simulink library "aerosimlib"  (Simulink 5.0)
values from neighbouring files (symbols this model uses):
  stdatm = [0 100 200 300 400 500 600 700 800 900 1000 1100 ... (4305 elements, 861x5)]    [stdatm.mat]
undefined symbols (not defined in the file or in its folder): AlphaBnd, b, BetaBnd, CDda, CDde, CDdf, CDdr, CDM, CDmin, CGempty, CGgross, CL0, CLa, CLalphadot, Clbeta, Clda, CLde, CLdf, Cldr, CLM, CLmind, Clp, CLq, Clr, Cm0, Cma, Cmalphadot, Cmde, Cmdf, CmM, Cmq, Cnbeta, Cnda, Cndr, Cnp, Cnr, CP, CT, CYbeta, CYda, CYdr, CYp, CYr, Displacement, dmy, Engine, EulerIni, FuelFlow, FuelIni, J, Jempty, Jeng, Jgross, Jprop, MAC, MAP, MAPLim, MassIni, MaxPower, mempty ... (+25)
libraries: aerosimlib x350, simulink3 x41
(part 7 of 10)

== system aerosimlib/FlightGear-Compatible/Complete Aircraft/CESSNA-182 ==
  Control : Inport  PortDimensions=[8 1]
  Wind : Inport  Port=2  PortDimensions=[3 1]
  RST : Inport  Port=3  PortDimensions=1
  Aerodynamics : Subsystem
  Aircraft Inertia : Subsystem
  Atmosphere : aerosimlib/FlightGear-Compatible/Complete Aircraft/CESSNA-172/Atmosphere  SimViewingDevice=off
      settings: Permissions=ReadWrite  RTWFcnNameOpts=Auto  RTWFileNameOpts=Auto
  Demux : Demux  Outputs=8
  Demux1 : Demux  Outputs=3
  Earth : Subsystem
  Equations of Motion : Subsystem
  F/m : Product  Inputs=*/  SaturateOnIntegerOverflow=on  InputSameDT=on
  FG Piston Engine +  Variable-Pitch Prop : aerosimlib/FlightGear-Compatible/Propulsion/FG Piston Engine +  Variable-Pitch Prop  Eng=AC.Propulsion.Engine{1}  Thr=AC.Propulsion.Thruster{1}  pSL=101325  TSL=288.15  OmegaIni=OmegaIni
  Mux : Mux
  Mux1 : Mux
  Sum1 : Sum  SaturateOnIntegerOverflow=on  InputSameDT=on
  Sum2 : Sum  SaturateOnIntegerOverflow=on  InputSameDT=on
  rad/s 2 RPM : aerosimlib/Unit Conversion/Angular velocity/rad//s 2 RPM
  TAS : Outport
  AOA : Outport  Port=2
  Position : Outport  Port=3
  Attitude : Outport  Port=4
  Rates : Outport  Port=5
  Aero : Outport  Port=6
  Prop : Outport  Port=7
  Engine : Outport  Port=8
  RPM : Outport  Port=9
  wires:
  Demux/8 -> Mux1/4
  rad/s 2 RPM/1 -> RPM/1
  FG Piston Engine +  Variable-Pitch Prop/3 -> rad/s 2 RPM/1
  FG Piston Engine +  Variable-Pitch Prop/5 -> Engine/1
  FG Piston Engine +  Variable-Pitch Prop/6 -> Prop/1
  Aerodynamics/3(AeroCoeff) -> Aero/1
  Equations of Motion/7(Euler) -> Attitude/1
  Demux1/3 -> AOA/1
  Demux1/1 -> TAS/1
  Equations of Motion/6(DCM) -> Atmosphere/6
  Equations of Motion/1(VelB) -> Aerodynamics/2(VelB), Atmosphere/4
  Equations of Motion/3(Rates) -> Rates/1, Aerodynamics/4(Rates)
  Earth/2(AGL) -> Aerodynamics/8(AGL), Atmosphere/2
  Earth/1(MSL) -> Atmosphere/1
  Earth/3(AConGnd) -> Equations of Motion/6(AConGnd)
  Earth/6(Gravity) -> Equations of Motion/5(Gravity)
  Earth/4(Rearth) -> Equations of Motion/4(Rearth)
  Equations of Motion/5(Pos) -> Position/1, Earth/1(Position)
  Aircraft Inertia/3(Inertia) -> Equations of Motion/3(Inertia)
  F/m/1 -> Equations of Motion/1(Accel)
  Aircraft Inertia/2(CG) -> FG Piston Engine +  Variable-Pitch Prop/6, Aerodynamics/9(CGpos)
  Aircraft Inertia/1(Mass) -> F/m/2
  FG Piston Engine +  Variable-Pitch Prop/4 -> Aircraft Inertia/1(FuelFlow)
  RST/1 -> Aircraft Inertia/2(RST), Equations of Motion/7(RST), FG Piston Engine +  Variable-Pitch Prop/7
  Aerodynamics/4(VelW) -> Demux1/1, FG Piston Engine +  Variable-Pitch Prop/5, Atmosphere/5
  Atmosphere/2 -> FG Piston Engine +  Variable-Pitch Prop/3
  Atmosphere/1 -> FG Piston Engine +  Variable-Pitch Prop/2
  Atmosphere/5 -> Aerodynamics/3(WindB)
  Atmosphere/6 -> Aerodynamics/5(WindRates)
  Wind/1 -> Atmosphere/3
  Atmosphere/4 -> Aerodynamics/7(a)
  Atmosphere/3 -> FG Piston Engine +  Variable-Pitch Prop/4, Aerodynamics/6(rho)
  Mux1/1 -> FG Piston Engine +  Variable-Pitch Prop/1
  Mux/1 -> Aerodynamics/1(Control)
  Control/1 -> Demux/1
  Demux/7 -> Mux1/3
  Demux/6 -> Mux1/2
  Demux/5 -> Mux1/1
  Demux/4 -> Mux/4
  Demux/3 -> Mux/3
  Demux/2 -> Mux/2
  Demux/1 -> Mux/1
  FG Piston Engine +  Variable-Pitch Prop/2 -> Sum1/2
  Sum2/1 -> F/m/1
  Sum1/1 -> Equations of Motion/2(Moment)
  Aerodynamics/1(Faero) -> Sum2/1
  Aerodynamics/2(Maero) -> Sum1/1
  FG Piston Engine +  Variable-Pitch Prop/1 -> Sum2/2

== system aerosimlib/FlightGear-Compatible/Complete Aircraft/CESSNA-310 ==
  Control : Inport  PortDimensions=[12 1]
  Gear : Inport  Port=2  PortDimensions=1
  Wind : Inport  Port=3  PortDimensions=[3 1]
  RST : Inport  Port=4  PortDimensions=1
  Aerodynamics : Subsystem
  Aircraft Inertia : Subsystem
  Atmosphere : aerosimlib/FlightGear-Compatible/Complete Aircraft/CESSNA-172/Atmosphere  SimViewingDevice=off
      settings: Permissions=ReadWrite  RTWFcnNameOpts=Auto  RTWFileNameOpts=Auto
  Demux : Demux  Outputs=3
  Demux1 : Demux  Outputs=3
  Earth : Subsystem
  Equations of Motion : Subsystem
  F/m : Product  Inputs=*/  SaturateOnIntegerOverflow=on  InputSameDT=on
  Left Engine : aerosimlib/FlightGear-Compatible/Propulsion/FG Piston Engine +  Variable-Pitch Prop  Eng=AC.Propulsion.Engine{1}  Thr=AC.Propulsion.Thruster{1}  pSL=101325  TSL=288.15  OmegaIni=OmegaIni(1)
  Right Engine : aerosimlib/FlightGear-Compatible/Propulsion/FG Piston Engine +  Variable-Pitch Prop  Eng=AC.Propulsion.Engine{2}  Thr=AC.Propulsion.Thruster{2}  pSL=101325  TSL=288.15  OmegaIni=OmegaIni(2)
  Sum : Sum  Orientation=left  Inputs=|++  SaturateOnIntegerOverflow=on  InputSameDT=on
  Sum1 : Sum  Inputs=+++  SaturateOnIntegerOverflow=on  InputSameDT=on
  Sum2 : Sum  Inputs=+++  SaturateOnIntegerOverflow=on  InputSameDT=on
  rad/s 2 RPM : aerosimlib/Unit Conversion/Angular velocity/rad//s 2 RPM
  rad/s 2 RPM1 : aerosimlib/Unit Conversion/Angular velocity/rad//s 2 RPM
  TAS : Outport
  AOA : Outport  Port=2
  Position : Outport  Port=3
  Attitude : Outport  Port=4
  Rates : Outport  Port=5
  Aero : Outport  Port=6
  PropL : Outport  Port=7
  EngineL : Outport  Port=8
  RPML : Outport  Port=9
  PropR : Outport  Port=10
  EngineR : Outport  Port=11
  RPMR : Outport  Port=12
  wires:
  Gear/1 -> Aerodynamics/10(Gear)
  Demux/1 -> Aerodynamics/1(Control)
  Earth/1(MSL) -> Atmosphere/1
  Equations of Motion/6(DCM) -> Atmosphere/6
  Earth/2(AGL) -> Aerodynamics/8(AGL), Atmosphere/2
  Atmosphere/4 -> Aerodynamics/7(a)
  Atmosphere/6 -> Aerodynamics/5(WindRates)
  Atmosphere/5 -> Aerodynamics/3(WindB)
  Equations of Motion/1(VelB) -> Aerodynamics/2(VelB), Atmosphere/4
  rad/s 2 RPM1/1 -> RPMR/1
  Right Engine/5 -> EngineR/1
  Right Engine/6 -> PropR/1
  rad/s 2 RPM/1 -> RPML/1
  Left Engine/6 -> PropL/1
  Left Engine/5 -> EngineL/1
  Right Engine/3 -> rad/s 2 RPM1/1
  Left Engine/3 -> rad/s 2 RPM/1
  Right Engine/2 -> Sum2/2
  Left Engine/2 -> Sum2/3
  Aerodynamics/2(Maero) -> Sum2/1
  Sum2/1 -> Equations of Motion/2(Moment)
  Right Engine/1 -> Sum1/2
  Left Engine/1 -> Sum1/3
  Aircraft Inertia/1(Mass) -> F/m/2
  Sum1/1 -> F/m/1
  F/m/1 -> Equations of Motion/1(Accel)
  Sum/1 -> Aircraft Inertia/1(FuelFlow)
  Left Engine/4 -> Sum/2
  Right Engine/4 -> Sum/1
  Atmosphere/3 -> Aerodynamics/6(rho), Right Engine/4, Left Engine/4
  Atmosphere/2 -> Right Engine/3, Left Engine/3
  Atmosphere/1 -> Right Engine/2, Left Engine/2
  Demux/3 -> Right Engine/1
  Demux/2 -> Left Engine/1
  Wind/1 -> Atmosphere/3
  Aerodynamics/3(AeroCoeff) -> Aero/1
  Equations of Motion/7(Euler) -> Attitude/1
  Demux1/3 -> AOA/1
  Demux1/1 -> TAS/1
  Equations of Motion/3(Rates) -> Rates/1, Aerodynamics/4(Rates)
  Earth/3(AConGnd) -> Equations of Motion/6(AConGnd)
  Earth/6(Gravity) -> Equations of Motion/5(Gravity)
  Earth/4(Rearth) -> Equations of Motion/4(Rearth)
  Equations of Motion/5(Pos) -> Position/1, Earth/1(Position)
  Aircraft Inertia/3(Inertia) -> Equations of Motion/3(Inertia)
  Aircraft Inertia/2(CG) -> Left Engine/6, Aerodynamics/9(CGpos), Right Engine/6
  Aerodynamics/1(Faero) -> Sum1/1
  RST/1 -> Right Engine/7, Left Engine/7, Aircraft Inertia/2(RST), Equations of Motion/7(RST)
  Aerodynamics/4(VelW) -> Right Engine/5, Left Engine/5, Atmosphere/5, Demux1/1
  Control/1 -> Demux/1

== system aerosimlib/FlightGear-Compatible/Inertia/Empty Aircraft ==
  ACMass : Constant  Value=Metrics.EmptyWeight
  CG Location : Constant  Value=Metrics.CGLoc
  Moments of Inertia : Constant  Value=[Metrics.InertiaX Metrics.InertiaY Metrics.InertiaZ Metrics.InertiaXZ]
  Mass : Outport
  CG : Outport  Port=2
  Inertia : Outport  Port=3
  wires:
  ACMass/1 -> Mass/1
  CG Location/1 -> CG/1
  Moments of Inertia/1 -> Inertia/1

== system aerosimlib/FlightGear-Compatible/Inertia/Point Mass ==
  J1 : Product  SaturateOnIntegerOverflow=on  InputSameDT=on
  J2 : Product  SaturateOnIntegerOverflow=on  InputSameDT=on
  J3 : Product  SaturateOnIntegerOverflow=on  InputSameDT=on
  Jxz : Product  Inputs=3  SaturateOnIntegerOverflow=on  InputSameDT=on
  M : Constant  Value=PointMass(1)
  Math Function1 : Math  Operator=square
  Math Function2 : Math  Operator=square
  Math Function3 : Math  Operator=square
  Mux : Mux  Inputs=3
  Mux1 : Mux
  Sum : Sum  SaturateOnIntegerOverflow=on  InputSameDT=on
  Sum1 : Sum  SaturateOnIntegerOverflow=on  InputSameDT=on
  Sum2 : Sum  SaturateOnIntegerOverflow=on  InputSameDT=on
  x pos : Constant  Value=PointMass(2)
  y pos : Constant  Value=PointMass(3)
  z pos : Constant  Value=PointMass(4)
  Mass : Outport
  CG : Outport  Port=2
  Inertia : Outport  Port=3
  wires:
  J3/1 -> Mux1/3
  J2/1 -> Mux1/2
  J1/1 -> Mux1/1
  Mux1/1 -> Inertia/1
  Jxz/1 -> Mux1/4
  Mux/1 -> CG/1
  Sum/1 -> J3/2
  Sum2/1 -> J2/2
  Sum1/1 -> J1/2
  Math Function3/1 -> Sum2/2, Sum1/2
  Math Function2/1 -> Sum1/1, Sum/2
  Math Function1/1 -> Sum2/1, Sum/1
  z pos/1 -> Math Function3/1, Mux/3, Jxz/3
  y pos/1 -> Mux/2, Math Function2/1
  x pos/1 -> Mux/1, Jxz/2, Math Function1/1
  M/1 -> Mass/1, J1/1, J2/1, J3/1, Jxz/1

== system aerosimlib/FlightGear-Compatible/Propulsion/Engine ==
  Piston : Subsystem

== system aerosimlib/FlightGear-Compatible/Propulsion/FG Piston Engine +  Fixed-Pitch Prop ==
  Control : Inport  PortDimensions=[3 1]  DataType=double
  p : Inport  Port=2  PortDimensions=1  DataType=double
  T : Inport  Port=3  PortDimensions=1  DataType=double
  rho : Inport  Port=4  PortDimensions=1  DataType=double
  WindAxesVel : Inport  Port=5  PortDimensions=[3 1]
  CGpos : Inport  Port=6  PortDimensions=[3 1]
  RST : Inport  Port=7  PortDimensions=1  DataType=double
  ChSign : Gain  Gain=-Thr.Sense  SaturateOnIntegerOverflow=on
  Demux : Demux  Outputs=3
  Demux1 : Demux  Outputs=3
  Engine speed Integrator : Integrator  ExternalReset=rising  InitialCondition=OmegaIni  LimitOutput=on  LowerSaturationLimit=0
  FG Fixed-Pitch Propeller : aerosimlib/FlightGear-Compatible/Propulsion/Thruster/Propeller/FG Fixed-Pitch Propeller  Thr=Thr
  FG Piston Engine : aerosimlib/FlightGear-Compatible/Propulsion/Engine/Piston/FG Piston Engine  Eng=Eng  pSL=pSL  TSL=TSL
  M/J : Product  Inputs=*/  SaturateOnIntegerOverflow=on  InputSameDT=on
  Mux : Mux  Inputs=3
  Mux1 : Mux  Inputs=3
  Mux2 : Mux  Inputs=5
  Propeller  moment of inertia : Constant  Value=Thr.Param.Inertia
  Sum : Sum  Inputs=|+-  SaturateOnIntegerOverflow=on  InputSameDT=on
  Sum1 : Sum  SaturateOnIntegerOverflow=on  InputSameDT=on
  Sum2 : Sum  Inputs=|++  SaturateOnIntegerOverflow=on  InputSameDT=on
  Terminator : Terminator
  Terminator1 : Terminator
  Zero : Constant  Value=0
  r x F : aerosimlib/Math/Cross Product
  r_prop : Constant  Value=Thr.Loc
  Fprop : Outport
  Mprop : Outport  Port=2
  Omega : Outport  Port=3
  FuelFlow : Outport  Port=4
  EngCoeff : Outport  Port=5
  PropCoeff : Outport  Port=6
  wires:
  Control/1 -> Demux/1
  WindAxesVel/1 -> Demux1/1
  Demux1/2 -> Terminator/1
  Demux1/3 -> Terminator1/1
  Demux1/1 -> FG Fixed-Pitch Propeller/1
  rho/1 -> FG Piston Engine/6, FG Fixed-Pitch Propeller/2
  Propeller  moment of inertia/1 -> M/J/2
  FG Fixed-Pitch Propeller/2 -> Sum1/2
  Sum1/1 -> M/J/1
  M/J/1 -> Engine speed Integrator/1
  RST/1 -> Engine speed Integrator/2
  Engine speed Integrator/1 -> FG Piston Engine/3, FG Fixed-Pitch Propeller/3, Omega/1
  Zero/1 -> Mux/2, Mux/3, Mux1/3, Mux1/2
  FG Fixed-Pitch Propeller/1 -> Mux/1
  ChSign/1 -> Mux1/1
  FG Fixed-Pitch Propeller/3 -> PropCoeff/1
  Demux/1 -> FG Piston Engine/1
  Demux/2 -> FG Piston Engine/2
  p/1 -> FG Piston Engine/4
  T/1 -> FG Piston Engine/5
  FG Piston Engine/6 -> ChSign/1, Sum1/1
  FG Piston Engine/1 -> Mux2/1
  FG Piston Engine/2 -> Mux2/2
  FG Piston Engine/3 -> Mux2/3, FuelFlow/1
  FG Piston Engine/4 -> Mux2/4
  FG Piston Engine/5 -> Mux2/5
  Mux2/1 -> EngCoeff/1
  r_prop/1 -> Sum/1
  CGpos/1 -> Sum/2
  Sum/1 -> r x F/1
  Mux/1 -> r x F/2, Fprop/1
  Mux1/1 -> Sum2/1
  r x F/1 -> Sum2/2
  Sum2/1 -> Mprop/1

== system aerosimlib/FlightGear-Compatible/Propulsion/FG Piston Engine +  Variable-Pitch Prop ==
  Control : Inport  PortDimensions=[4 1]  DataType=double
  p : Inport  Port=2  PortDimensions=1  DataType=double
  T : Inport  Port=3  PortDimensions=1  DataType=double
  rho : Inport  Port=4  PortDimensions=1  DataType=double
  WindAxesVel : Inport  Port=5  PortDimensions=[3 1]
  CGpos : Inport  Port=6  PortDimensions=[3 1]
  RST : Inport  Port=7  PortDimensions=1  DataType=double
  ChSign : Gain  Gain=-Thr.Sense  SaturateOnIntegerOverflow=on
  Demux : Demux
  Demux1 : Demux  Outputs=3
  Engine speed Integrator : Integrator  ExternalReset=rising  InitialCondition=OmegaIni  LimitOutput=on  LowerSaturationLimit=0
  FG Piston Engine : aerosimlib/FlightGear-Compatible/Propulsion/Engine/Piston/FG Piston Engine  Eng=Eng  pSL=pSL  TSL=TSL
  FG Variable-Pitch Propeller : aerosimlib/FlightGear-Compatible/Propulsion/Thruster/Propeller/FG Variable-Pitch Propeller  Thr=Thr
  M/J : Product  Inputs=*/  SaturateOnIntegerOverflow=on  InputSameDT=on
  Mux : Mux  Inputs=3
  Mux1 : Mux  Inputs=3
  Mux2 : Mux  Inputs=5
  Propeller  moment of inertia : Constant  Value=Thr.Param.Inertia
  Sum : Sum  Inputs=|+-  SaturateOnIntegerOverflow=on  InputSameDT=on
  Sum1 : Sum  SaturateOnIntegerOverflow=on  InputSameDT=on
  Sum2 : Sum  Inputs=|++  SaturateOnIntegerOverflow=on  InputSameDT=on
  Terminator : Terminator
  Terminator1 : Terminator
  Zero : Constant  Value=0
  r x F : aerosimlib/Math/Cross Product
  r_prop : Constant  Value=Thr.Loc
  Fprop : Outport
  Mprop : Outport  Port=2
  Omega : Outport  Port=3
  FuelFlow : Outport  Port=4
  EngCoeff : Outport  Port=5
  PropCoeff : Outport  Port=6
  wires:
  Demux/4 -> FG Variable-Pitch Propeller/4
  Control/1 -> Demux/1
  WindAxesVel/1 -> Demux1/1
  Demux1/2 -> Terminator/1
  Demux1/3 -> Terminator1/1
  Demux1/1 -> FG Variable-Pitch Propeller/1
  rho/1 -> FG Variable-Pitch Propeller/2, FG Piston Engine/6
  Propeller  moment of inertia/1 -> M/J/2
  FG Variable-Pitch Propeller/2 -> Sum1/2
  Sum1/1 -> M/J/1
  M/J/1 -> Engine speed Integrator/1
  RST/1 -> Engine speed Integrator/2
  Engine speed Integrator/1 -> FG Variable-Pitch Propeller/3, FG Piston Engine/3, Omega/1
  Zero/1 -> Mux/2, Mux/3, Mux1/3, Mux1/2
  FG Variable-Pitch Propeller/1 -> Mux/1
  ChSign/1 -> Mux1/1
  FG Variable-Pitch Propeller/3 -> PropCoeff/1
  Demux/1 -> FG Piston Engine/1
  Demux/2 -> FG Piston Engine/2
  p/1 -> FG Piston Engine/4
  T/1 -> FG Piston Engine/5
  FG Piston Engine/6 -> ChSign/1, Sum1/1
  FG Piston Engine/1 -> Mux2/1
  FG Piston Engine/2 -> Mux2/2
  FG Piston Engine/3 -> Mux2/3, FuelFlow/1
  FG Piston Engine/4 -> Mux2/4
  FG Piston Engine/5 -> Mux2/5
  Mux2/1 -> EngCoeff/1
  r_prop/1 -> Sum/1
  CGpos/1 -> Sum/2
  Sum/1 -> r x F/1
  Mux/1 -> r x F/2, Fprop/1
  Mux1/1 -> Sum2/1
  r x F/1 -> Sum2/2
  Sum2/1 -> Mprop/1

== system aerosimlib/FlightGear-Compatible/Propulsion/Tank ==
  Fuel Tank : Subsystem  mask(Fuel Tank){MassIni=MassIni, Tank=Tank}
      mask prompts: MassIni "Initial mass:"; Tank "Tank structure:"
      mask help: The block integrates fuel flow to compute the tank inertia parameters.
      mask init:
      | if MassIni > Tank.Capacity
      | 	% Limit initial mass to tank capacity
      | 	MassIni = Tank.Capacity;
      | end
      mask Help:
      | The block integrates fuel flow to compute the tank inertia parameters.
      | <P><B>Inputs:</B>
      | <LI>MassFlow = the current propellant mass flow (positive for propellant flowing out of the tank, negative otherwise)</LI>
      | <LI>RST = the flow integrator reset flag (integrator resets on rising edge)</LI>
      | </P>
      | <P><B>Outputs:</B>
      | <LI>Mass = the current mass of the propellant in the tank</LI>
      | <LI>CG = the tank CG location, in aircraft coordinates</LI>
      | <LI>Inertia = the tank moments of inertia [Jx Jy Jz Jxz]</LI>
      | </P>
      | <P><B>Parameters:</B>
      | <LI>Initial mass = the initial mass of propellant in the tank</LI>
      | <LI>Tank structure = the Matlab tank structure, part of the aircraft structure</LI>
      | </P>

== system aerosimlib/FlightGear-Compatible/Propulsion/Thruster ==
  Propeller : Subsystem

== system aerosimlib/Math/Normalization/Vector norm ==
  Vec : Inport
  Dot Product : simulink3/Math/Dot Product
  Math Function : Math  Operator=sqrt
  Mag : Outport
  wires:
  Math Function/1 -> Mag/1
  Dot Product/1 -> Math Function/1
  Vec/1 -> Dot Product/2, Dot Product/1

== system aerosimlib/Math/Zero Offset/Non-zero Sign ==
  In : Inport
  One : Constant
  Relational Operator : RelationalOperator  Operator===  InputSameDT=on
  Sign : Signum
  Switch : Switch  Threshold=1  SaturateOnIntegerOverflow=on  InputSameDT=on
  Zero : Constant  Value=0
  Out : Outport
  wires:
  Zero/1 -> Relational Operator/2
  In/1 -> Relational Operator/1, Sign/1
  Relational Operator/1 -> Switch/2
  One/1 -> Switch/1
  Sign/1 -> Switch/3
  Switch/1 -> Out/1

== system aerosimlib/Propulsion/Piston Engine/Intake ==
  Thr : Inport  PortDimensions=1  DataType=double
  p : Inport  Port=2  PortDimensions=1  DataType=double
  Get MAP : Product  SaturateOnIntegerOverflow=on  InputSameDT=on
  MAP min : Constant  Value=MAPmin
  Saturation : Saturate  UpperLimit=inf  LowerLimit=MAPmin
  Sum : Sum  Inputs=|+-  SaturateOnIntegerOverflow=on  InputSameDT=on
  Sum1 : Sum  Inputs=|++  SaturateOnIntegerOverflow=on  InputSameDT=on
  kPa : Gain  Gain=1/1000  SaturateOnIntegerOverflow=on
  MAP : Outport
  wires:
  Saturation/1 -> MAP/1
  p/1 -> kPa/1
  Thr/1 -> Get MAP/1
  MAP min/1 -> Sum/2, Sum1/2
  kPa/1 -> Sum/1
  Sum/1 -> Get MAP/2
  Get MAP/1 -> Sum1/1
  Sum1/1 -> Saturation/1

== system aerosimlib/Sensors/Analog Sensors/A/D Converter ==
  Analog : Inport
  Count size in Volts : Product  Inputs=*/  SaturateOnIntegerOverflow=on  InputSameDT=on
  Max Counts : Constant  Value=2^Bits
  Max Volts : Constant  Value=MaxVolts
  Min Volts : Constant  Value=MinVolts
  Number of counts : Product  Inputs=*/  SaturateOnIntegerOverflow=on  InputSameDT=on
  Rounding Function : Rounding
  Saturation : Saturate  UpperLimit=2^Bits  LowerLimit=0
  Sum : Sum  Inputs=|+-  SaturateOnIntegerOverflow=on  InputSameDT=on
  Sum1 : Sum  Inputs=|+-  SaturateOnIntegerOverflow=on  InputSameDT=on
  Zero-Order Hold : ZeroOrderHold  SampleTime=tsamp
  Digital : Outport
  wires:
  Zero-Order Hold/1 -> Digital/1
  Saturation/1 -> Zero-Order Hold/1
  Max Volts/1 -> Sum/1
  Min Volts/1 -> Sum/2, Sum1/2
  Max Counts/1 -> Count size in Volts/2
  Sum/1 -> Count size in Volts/1
  Analog/1 -> Sum1/1
  Sum1/1 -> Number of counts/1
  Count size in Volts/1 -> Number of counts/2
  Number of counts/1 -> Rounding Function/1
  Rounding Function/1 -> Saturation/1

== system aerosimlib/Sensors/Analog Sensors/Analog Sensor ==
  Input : Inport  PortDimensions=1
  Bias Voltage : Constant  Value=BiasVolt
  Bias Point : Constant  Value=BiasPoint
  Scale Factor : Constant  Value=ScaleFactor
  Simple Sensor (2nd-order dynamics) : aerosimlib/Sensors/Generic Sensors/Simple Sensor (2nd-order dynamics)  MaxInput=Range(2)  MinInput=Range(1)  Bandwidth=Bandwidth  NoiseSeed=NoiseSeed  NoiseCov=NoiseCov  SampleTime=SampleTime
  Sum1 : Sum  Inputs=|++  SaturateOnIntegerOverflow=on  InputSameDT=on
  Sum2 : Sum  Inputs=|+-  SaturateOnIntegerOverflow=on  InputSameDT=on
  Unit conversion : Product  SaturateOnIntegerOverflow=on  InputSameDT=on
  Output : Outport
  wires:
  Simple Sensor (2nd-order dynamics)/1 -> Sum2/1
  Bias Point/1 -> Sum2/2
  Sum2/1 -> Unit conversion/1
  Scale Factor/1 -> Unit conversion/2
  Unit conversion/1 -> Sum1/1
  Bias Voltage/1 -> Sum1/2
  Sum1/1 -> Output/1
  Input/1 -> Simple Sensor (2nd-order dynamics)/1

== system aerosimlib/Sensors/Digital Sensors/GPS PV ==
  PVIn : Inport
  Altitude Measurement : aerosimlib/Sensors/Digital Sensors/Single GPS Measurement  ValIni=PosIni(3)  Lag=PosLag  TimeConst=TimeConst  seed=[32214]  Cov=VPosErr  T1=Trw
  Demux : Demux  Outputs=6
  Latitude Measurement : aerosimlib/Sensors/Digital Sensors/Single GPS Measurement  ValIni=PosIni(1)  Lag=PosLag  TimeConst=TimeConst  seed=[44123]  Cov=HPosErr/REarth  T1=Trw
  Longitude Measurement : aerosimlib/Sensors/Digital Sensors/Single GPS Measurement  ValIni=PosIni(2)  Lag=PosLag  TimeConst=TimeConst  seed=[11243]  Cov=HPosErr/REarth  T1=Trw
  Mux : Mux  Inputs=6
  V Down Measurement : aerosimlib/Sensors/Digital Sensors/Single GPS Measurement  ValIni=VelIni(3)  Lag=VelLag  TimeConst=TimeConst  seed=[21143]  Cov=VVelErr  T1=Trw
  V East Measurement : aerosimlib/Sensors/Digital Sensors/Single GPS Measurement  ValIni=VelIni(2)  Lag=VelLag  TimeConst=TimeConst  seed=[43321]  Cov=HVelErr  T1=Trw
  V North Measurement : aerosimlib/Sensors/Digital Sensors/Single GPS Measurement  ValIni=VelIni(1)  Lag=VelLag  TimeConst=TimeConst  seed=[12344]  Cov=HVelErr  T1=Trw
  PVOut : Outport
  wires:
  Demux/1 -> Latitude Measurement/1
  Demux/2 -> Longitude Measurement/1
  Demux/3 -> Altitude Measurement/1
  Demux/4 -> V North Measurement/1
  Demux/5 -> V East Measurement/1
  Demux/6 -> V Down Measurement/1
  PVIn/1 -> Demux/1
  Latitude Measurement/1 -> Mux/1
  Longitude Measurement/1 -> Mux/2
  Altitude Measurement/1 -> Mux/3
  V North Measurement/1 -> Mux/4
  V East Measurement/1 -> Mux/5
  V Down Measurement/1 -> Mux/6
  Mux/1 -> PVOut/1

== system aerosimlib/Sensors/Digital Sensors/Single GPS Measurement ==
  In : Inport
  Gauss-Markov  Process : aerosimlib/Sensors/Noise Correlation/Gauss-Markov  Process  beta=TimeConst  seed=seed  Var=Cov^2  T=T1
  Sum : Sum  Inputs=|++  SaturateOnIntegerOverflow=on  InputSameDT=on
  Transport Delay : TransportDelay  DelayTime=Lag  InitialInput=ValIni
  Out : Outport
  wires:
  Sum/1 -> Out/1
  Gauss-Markov  Process/1 -> Sum/2
  In/1 -> Transport Delay/1
  Transport Delay/1 -> Sum/1

== system aerosimlib/Sensors/Generic Sensors/Simple Sensor (1st-order dynamics) ==
  Input : Inport
  Random Walk : aerosimlib/Sensors/Noise Correlation/Random Walk  seed=NoiseSeed  Var=NoiseCov  T=SampleTime
  Saturation : Saturate  UpperLimit=MaxInput  LowerLimit=MinInput
  Sum : Sum  Inputs=|++  SaturateOnIntegerOverflow=on  InputSameDT=on
  Transfer Fcn : TransferFcn  Denominator=[Lag 1]
  Output : Outport
  wires:
  Sum/1 -> Output/1
  Random Walk/1 -> Sum/2
  Transfer Fcn/1 -> Sum/1
  Saturation/1 -> Transfer Fcn/1
  Input/1 -> Saturation/1

== system aerosimlib/Sensors/Generic Sensors/Simple Sensor (2nd-order dynamics) ==
  Input : Inport
  Random Walk : aerosimlib/Sensors/Noise Correlation/Random Walk  seed=NoiseSeed  Var=NoiseCov  T=SampleTime
  Saturation : Saturate  UpperLimit=MaxInput  LowerLimit=MinInput
  Sum : Sum  Inputs=|++  SaturateOnIntegerOverflow=on  InputSameDT=on
  Transfer Fcn : TransferFcn  Numerator=[wn^2]  Denominator=[1 2*zeta*wn wn^2]
  Output : Outport
  wires:
  Input/1 -> Saturation/1
  Saturation/1 -> Transfer Fcn/1
  Transfer Fcn/1 -> Sum/1
  Random Walk/1 -> Sum/2
  Sum/1 -> Output/1

== system aerosimlib/Sensors/Noise Correlation/Gauss-Markov  Process ==
  Gain : Gain  Orientation=left  Gain=1/beta  SaturateOnIntegerOverflow=on
  Integrator : Integrator
  Sum : Sum  Inputs=|+-  SaturateOnIntegerOverflow=on  InputSameDT=on
  White Noise : RandomNumber  Variance=Var  Seed=seed  SampleTime=T
  Out : Outport
  wires:
  Integrator/1 -> Out/1, Gain/1
  White Noise/1 -> Sum/1
  Sum/1 -> Integrator/1
  Gain/1 -> Sum/2

== system aerosimlib/Sensors/Noise Correlation/Random Walk ==
  Integrator : Integrator
  White Noise : RandomNumber  Variance=Var  Seed=seed  SampleTime=T
  Out : Outport
  wires:
  White Noise/1 -> Integrator/1
  Integrator/1 -> Out/1

== system aerosimlib/Unit Conversion/Angular position/deg 2 rad ==
  In : Inport
  Gain : Gain  Gain=pi/180  SaturateOnIntegerOverflow=on
  Out : Outport
  wires:
  Gain/1 -> Out/1
  In/1 -> Gain/1

== system aerosimlib/Unit Conversion/Angular position/rad 2 deg ==
  In : Inport
  Gain : Gain  Gain=180/pi  SaturateOnIntegerOverflow=on
  Out : Outport
  wires:
  In/1 -> Gain/1
  Gain/1 -> Out/1

== system aerosimlib/Unit Conversion/Angular velocity/RPM 2 rad/s ==
  In : Inport
  Gain : Gain  Gain=pi/30  SaturateOnIntegerOverflow=on
  Out : Outport
  wires:
  In/1 -> Gain/1
  Gain/1 -> Out/1

== system aerosimlib/Unit Conversion/Angular velocity/rad/s 2 RPM ==
  In : Inport
  Gain : Gain  Gain=30/pi  SaturateOnIntegerOverflow=on
  Out : Outport
  wires:
  Gain/1 -> Out/1
  In/1 -> Gain/1

== system aerosimlib/Unit Conversion/Distance/ft 2 m ==
  In : Inport
  Gain : Gain  Gain=0.3048  SaturateOnIntegerOverflow=on
  Out : Outport
  wires:
  In/1 -> Gain/1
  Gain/1 -> Out/1

== system aerosimlib/Unit Conversion/Distance/m 2 ft ==
  In : Inport
  Gain : Gain  Gain=1/0.3048  SaturateOnIntegerOverflow=on
  Out : Outport
  wires:
  Gain/1 -> Out/1
  In/1 -> Gain/1

== system aerosimlib/Unit Conversion/Distance/m 2 nm ==
  In : Inport
  Gain : Gain  Gain=1/1853.24496  SaturateOnIntegerOverflow=on
  Out : Outport
  wires:
  In/1 -> Gain/1
  Gain/1 -> Out/1

== system aerosimlib/Unit Conversion/Distance/nm 2 m ==
  In : Inport
  Gain : Gain  Gain=1853.24496  SaturateOnIntegerOverflow=on
  Out : Outport
  wires:
  Gain/1 -> Out/1
  In/1 -> Gain/1

== system aerosimlib/Unit Conversion/Force/N 2 lbf ==
  In : Inport
  Gain : Gain  Gain=0.22481  SaturateOnIntegerOverflow=on
  Out : Outport
  wires:
  Gain/1 -> Out/1
  In/1 -> Gain/1

== system aerosimlib/Unit Conversion/Force/lbf 2 N ==
  In : Inport
  Gain : Gain  Gain=1/0.22481  SaturateOnIntegerOverflow=on
  Out : Outport
  wires:
  In/1 -> Gain/1
  Gain/1 -> Out/1

== system aerosimlib/Unit Conversion/Mass/kg 2 lb ==
  In : Inport
  Gravity : Inport  Port=2
  Gain : Gain  Gain=0.22481  SaturateOnIntegerOverflow=on
  Product : Product  SaturateOnIntegerOverflow=on  InputSameDT=on
  Out : Outport
  wires:
  Product/1 -> Gain/1
  Gravity/1 -> Product/2
  In/1 -> Product/1
  Gain/1 -> Out/1

== system aerosimlib/Unit Conversion/Mass/kg 2 slug ==
  In : Inport
  Gain : Gain  Gain=0.068521  SaturateOnIntegerOverflow=on
  Out : Outport
  wires:
  In/1 -> Gain/1
  Gain/1 -> Out/1

== system aerosimlib/Unit Conversion/Mass/lb 2 kg ==
  In : Inport
  Gravity : Inport  Port=2
  Gain : Gain  Gain=1/0.22481  SaturateOnIntegerOverflow=on
  Product : Product  Inputs=*/  SaturateOnIntegerOverflow=on  InputSameDT=on
  Out : Outport
  wires:
  Product/1 -> Gain/1
  Gravity/1 -> Product/2
  In/1 -> Product/1
  Gain/1 -> Out/1

== system aerosimlib/Unit Conversion/Mass/slug 2 kg ==
  In : Inport
  Gain : Gain  Gain=1/0.068521  SaturateOnIntegerOverflow=on
  Out : Outport
  wires:
  Gain/1 -> Out/1
  In/1 -> Gain/1

== system aerosimlib/Unit Conversion/Pressure/Pa2inHg ==
  Pa : Inport
  Gain : Gain  Gain=0.00029529  SaturateOnIntegerOverflow=on
  inHg : Outport
  wires:
  Gain/1 -> inHg/1
  Pa/1 -> Gain/1

== system aerosimlib/Unit Conversion/Pressure/inHg2Pa ==
  inHg : Inport
  Gain : Gain  Gain=1/0.00029529  SaturateOnIntegerOverflow=on
  Pa : Outport
  wires:
  inHg/1 -> Gain/1
  Gain/1 -> Pa/1

== system aerosimlib/Unit Conversion/Temperature/F2K ==
  F : Inport
  Constant : Constant  Value=459.67
  Gain : Gain  Gain=1/1.8  SaturateOnIntegerOverflow=on
  Sum : Sum  Inputs=|++  SaturateOnIntegerOverflow=on  InputSameDT=on
  K : Outport
  wires:
  Constant/1 -> Sum/2
  F/1 -> Sum/1
  Sum/1 -> Gain/1
  Gain/1 -> K/1

== system aerosimlib/Unit Conversion/Temperature/K2F ==
  K : Inport
  Constant : Constant  Value=459.67
  Gain : Gain  Gain=1.8  SaturateOnIntegerOverflow=on
  Sum : Sum  Inputs=|+-  SaturateOnIntegerOverflow=on  InputSameDT=on
  F : Outport
  wires:
  K/1 -> Gain/1
  Gain/1 -> Sum/1
  Constant/1 -> Sum/2
  Sum/1 -> F/1

== system aerosimlib/Unit Conversion/Velocity/km/h 2 m/s ==
  In : Inport
  Gain : Gain  Gain=1/3.6  SaturateOnIntegerOverflow=on
  Out : Outport
  wires:
  Gain/1 -> Out/1
  In/1 -> Gain/1

== system aerosimlib/Unit Conversion/Velocity/kts 2 m/s ==
  In : Inport
  Gain : Gain  Gain=0.5147902667  SaturateOnIntegerOverflow=on
  Out : Outport
  wires:
  Gain/1 -> Out/1
  In/1 -> Gain/1

== system aerosimlib/Unit Conversion/Velocity/m/s 2 km/h ==
  In : Inport
  Gain : Gain  Gain=3.6  SaturateOnIntegerOverflow=on
  Out : Outport
  wires:
  In/1 -> Gain/1
  Gain/1 -> Out/1

== system aerosimlib/Unit Conversion/Velocity/m/s 2 kts ==
  In : Inport
  Gain : Gain  Gain=1.9425386701  SaturateOnIntegerOverflow=on
  Out : Outport
  wires:
  In/1 -> Gain/1
  Gain/1 -> Out/1

== system aerosimlib/Unit Conversion/Velocity/m/s 2 mph ==
  In : Inport
  Gain : Gain  Gain=2.2369362921  SaturateOnIntegerOverflow=on
  Out : Outport
  wires:
  Gain/1 -> Out/1
  In/1 -> Gain/1

== system aerosimlib/Unit Conversion/Velocity/mph 2 m/s ==
  In : Inport
  Gain : Gain  Gain=0.44704  SaturateOnIntegerOverflow=on
  Out : Outport
  wires:
  In/1 -> Gain/1
  Gain/1 -> Out/1

== system aerosimlib/Unit Conversion/Volume/gal 2 l ==
  In : Inport
  Gain : Gain  Gain=3.785412  SaturateOnIntegerOverflow=on
  Out : Outport
  wires:
  Gain/1 -> Out/1
  In/1 -> Gain/1

== system aerosimlib/Unit Conversion/Volume/l 2 gal ==
  In : Inport
  Gain : Gain  Gain=1/3.785412  SaturateOnIntegerOverflow=on
  Out : Outport
  wires:
  In/1 -> Gain/1
  Gain/1 -> Out/1

== system aerosimlib/Atmosphere/Turbulence/Turbulence Characteristics/Vector norm ==
  Vec : Inport
  Dot Product : simulink3/Math/Dot Product
  Math Function : Math  Operator=sqrt
  Mag : Outport
  wires:
  Vec/1 -> Dot Product/1, Dot Product/2
  Dot Product/1 -> Math Function/1
  Math Function/1 -> Mag/1

== system aerosimlib/Atmosphere/Wind Shear/Zero Offset1/Non-zero Sign ==
  In : Inport
  One : Constant
  Relational Operator : RelationalOperator  Operator===  InputSameDT=on
  Sign : Signum
  Switch : Switch  Threshold=1  SaturateOnIntegerOverflow=on  InputSameDT=on
  Zero : Constant  Value=0
  Out : Outport
  wires:
  Zero/1 -> Relational Operator/2
  In/1 -> Relational Operator/1, Sign/1
  Relational Operator/1 -> Switch/2
  One/1 -> Switch/1
  Sign/1 -> Switch/3
  Switch/1 -> Out/1

== system aerosimlib/Atmosphere/Wind Shear/Zero Offset2/Non-zero Sign ==
  In : Inport
  One : Constant
  Relational Operator : RelationalOperator  Operator===  InputSameDT=on
  Sign : Signum
  Switch : Switch  Threshold=1  SaturateOnIntegerOverflow=on  InputSameDT=on
  Zero : Constant  Value=0
  Out : Outport
  wires:
  Switch/1 -> Out/1
  Sign/1 -> Switch/3
  One/1 -> Switch/1
  Relational Operator/1 -> Switch/2
  In/1 -> Sign/1, Relational Operator/1
  Zero/1 -> Relational Operator/2

== system aerosimlib/Equations of Motion/Body-Frame EOM/Kinematics (Quaternions)/Normalization ==
  VecIn : Inport
  Vector norm : Subsystem
      mask Type: Vector norm-2
      mask Description: Compute the 2-norm (magnitude) of a vector, |v| = sqrt(v'v)
  e/|e| : Product  Inputs=*/  SaturateOnIntegerOverflow=on  InputSameDT=on
  VecOut : Outport
  wires:
  Vector norm/1(Mag) -> e/|e|/2
  e/|e|/1 -> VecOut/1
  VecIn/1 -> Vector norm/1(Vec), e/|e|/1

== system aerosimlib/Equations of Motion/Body-Frame EOM/Navigation/Latitude Bound ==
  In : Inport
  2pi : Constant  Value=2*pi
  ChSign : Gain  Gain=-1  SaturateOnIntegerOverflow=on
  Math Function : Math  Operator=mod
  Math Function1 : Math  Operator=mod
  Sum1 : Sum  Inputs=|+-  SaturateOnIntegerOverflow=on  InputSameDT=on
  Sum2 : Sum  Inputs=|++  SaturateOnIntegerOverflow=on  InputSameDT=on
  Switch : Switch  Threshold=pi  SaturateOnIntegerOverflow=on  InputSameDT=on
  pi : Constant  Value=pi
  pi/2 : Constant  Value=pi/2
  Out : Outport
  wires:
  2pi/1 -> Math Function1/2
  ChSign/1 -> Switch/1
  Sum2/1 -> Math Function1/1, Math Function/1
  In/1 -> Sum2/1
  Switch/1 -> Out/1
  Math Function1/1 -> Switch/2
  Sum1/1 -> Switch/3, ChSign/1
  pi/2/1 -> Sum2/2, Sum1/2
  Math Function/1 -> Sum1/1
  pi/1 -> Math Function/2

== system aerosimlib/Equations of Motion/Body-Frame EOM/Navigation/Longitude Bound ==
  In : Inport
  2pi : Constant  Value=2*pi
  Math Function : Math  Operator=mod
  Sum1 : Sum  Inputs=|+-  SaturateOnIntegerOverflow=on  InputSameDT=on
  Sum2 : Sum  Inputs=|++  SaturateOnIntegerOverflow=on  InputSameDT=on
  pi : Constant  Value=pi
  Out : Outport
  wires:
  Math Function/1 -> Sum1/1
  2pi/1 -> Math Function/2
  In/1 -> Sum2/1
  Sum2/1 -> Math Function/1
  pi/1 -> Sum2/2, Sum1/2
  Sum1/1 -> Out/1

== system aerosimlib/Equations of Motion/Geodetic-Frame EOM/Position/Latitude Bound ==
  In : Inport
  2pi : Constant  Value=2*pi
  ChSign : Gain  Gain=-1  SaturateOnIntegerOverflow=on
  Math Function : Math  Operator=mod
  Math Function1 : Math  Operator=mod
  Sum1 : Sum  Inputs=|+-  SaturateOnIntegerOverflow=on  InputSameDT=on
  Sum2 : Sum  Inputs=|++  SaturateOnIntegerOverflow=on  InputSameDT=on
  Switch : Switch  Threshold=pi  SaturateOnIntegerOverflow=on  InputSameDT=on
  pi : Constant  Value=pi
  pi/2 : Constant  Value=pi/2
  Out : Outport
  wires:
  pi/1 -> Math Function/2
  Math Function/1 -> Sum1/1
  pi/2/1 -> Sum1/2, Sum2/2
  Sum1/1 -> ChSign/1, Switch/3
  Math Function1/1 -> Switch/2
  Switch/1 -> Out/1
  In/1 -> Sum2/1
  Sum2/1 -> Math Function/1, Math Function1/1
  ChSign/1 -> Switch/1
  2pi/1 -> Math Function1/2

== system aerosimlib/Equations of Motion/Geodetic-Frame EOM/Position/Longitude Bound ==
  In : Inport
  2pi : Constant  Value=2*pi
  Math Function : Math  Operator=mod
  Sum1 : Sum  Inputs=|+-  SaturateOnIntegerOverflow=on  InputSameDT=on
  Sum2 : Sum  Inputs=|++  SaturateOnIntegerOverflow=on  InputSameDT=on
  pi : Constant  Value=pi
  Out : Outport
  wires:
  Sum1/1 -> Out/1
  pi/1 -> Sum1/2, Sum2/2
  Sum2/1 -> Math Function/1
  In/1 -> Sum2/1
  2pi/1 -> Math Function/2
  Math Function/1 -> Sum1/1

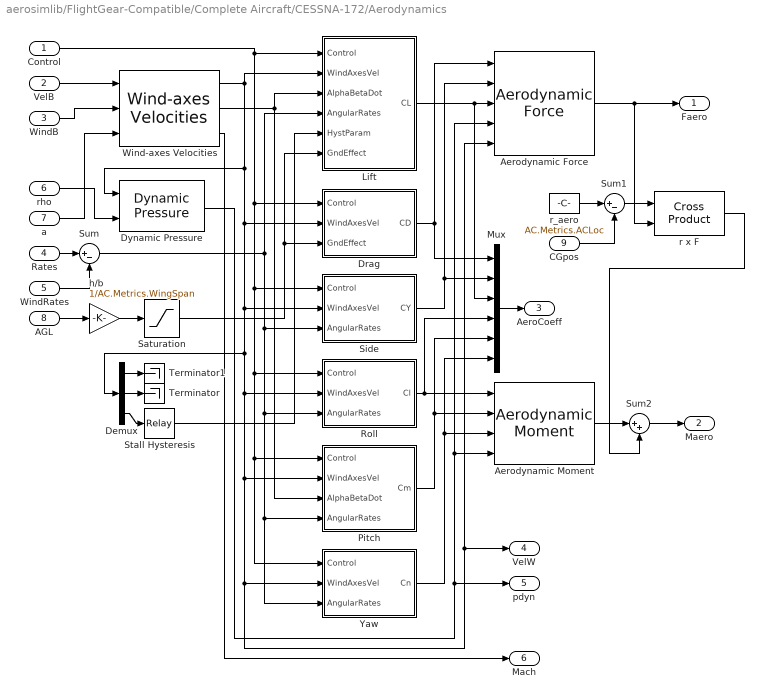
== system aerosimlib/FlightGear-Compatible/Complete Aircraft/CESSNA-172/Aerodynamics ==
  Control : Inport  PortDimensions=[4 1]
  VelB : Inport  Port=2  PortDimensions=[3 1]
  WindB : Inport  Port=3  PortDimensions=[3 1]
  Rates : Inport  Port=4  PortDimensions=[3 1]
  WindRates : Inport  Port=5  PortDimensions=[3 1]
  rho : Inport  Port=6  PortDimensions=1
  a : Inport  Port=7  PortDimensions=1
  AGL : Inport  Port=8  PortDimensions=1
  CGpos : Inport  Port=9  PortDimensions=[3 1]
  Aerodynamic Force : aerosimlib/Aerodynamics/Aerodynamic Force  S=AC.Metrics.WingArea
  Aerodynamic Moment : aerosimlib/Aerodynamics/Aerodynamic Moment  c=AC.Metrics.WingChord  b=AC.Metrics.WingSpan  S=AC.Metrics.WingArea
  Demux : Demux  Outputs=3
  Drag : Subsystem
  Dynamic Pressure : aerosimlib/Aerodynamics/Dynamic Pressure
  Lift : Subsystem
  Mux : Mux  Inputs=6
  Pitch : Subsystem
  Roll : Subsystem
  Saturation : Saturate  UpperLimit=1  LowerLimit=0
  Side : Subsystem
  Stall Hysteresis : Relay  OnSwitchValue=AC.Aerodynamics.HystLim(2)  OffSwitchValue=AC.Aerodynamics.HystLim(1)
  Sum : Sum  Inputs=|+-  SaturateOnIntegerOverflow=on  InputSameDT=on
  Sum1 : Sum  Inputs=|+-  SaturateOnIntegerOverflow=on  InputSameDT=on
  Sum2 : Sum  Inputs=|++  SaturateOnIntegerOverflow=on  InputSameDT=on
  Terminator : Terminator
  Terminator1 : Terminator
  Wind-axes Velocities : aerosimlib/Aerodynamics/Wind-axes Velocities  Vabnd=[0 1000]  betabnd=[-1 1]  alphabnd=AC.Aerodynamics.AlphaLim
  Yaw : Subsystem
  h/b : Gain  Gain=1/AC.Metrics.WingSpan  SaturateOnIntegerOverflow=on
  r x F : aerosimlib/Math/Cross Product
  r_aero : Constant  Value=AC.Metrics.ACLoc
  Faero : Outport
  Maero : Outport  Port=2
  AeroCoeff : Outport  Port=3
  VelW : Outport  Port=4
  pdyn : Outport  Port=5
  Mach : Outport  Port=6
  wires:
  Sum/1 -> Yaw/3(AngularRates), Pitch/4(AngularRates), Roll/3(AngularRates), Side/3(AngularRates), Lift/4(AngularRates)
  WindRates/1 -> Sum/2
  Rates/1 -> Sum/1
  Stall Hysteresis/1 -> Lift/5(HystParam)
  Demux/2 -> Terminator/1
  Demux/1 -> Terminator1/1
  Demux/3 -> Stall Hysteresis/1
  Saturation/1 -> Drag/3(GndEffect), Lift/6(GndEffect)
  AGL/1 -> h/b/1
  h/b/1 -> Saturation/1
  Wind-axes Velocities/3 -> Mach/1
  Yaw/1(Cn) -> Mux/6, Aerodynamic Moment/3
  Pitch/1(Cm) -> Mux/5, Aerodynamic Moment/2
  Roll/1(Cl) -> Mux/4, Aerodynamic Moment/1
  Dynamic Pressure/1 -> pdyn/1, Aerodynamic Moment/4, Aerodynamic Force/4
  Side/1(CY) -> Mux/2, Aerodynamic Force/2
  Drag/1(CD) -> Mux/1, Aerodynamic Force/1
  Lift/1(CL) -> Mux/3, Aerodynamic Force/3
  Wind-axes Velocities/2 -> Lift/3(AlphaBetaDot), Pitch/3(AlphaBetaDot)
  Control/1 -> Pitch/1(Control), Yaw/1(Control), Roll/1(Control), Side/1(Control), Drag/1(Control), Lift/1(Control)
  Wind-axes Velocities/1 -> Lift/2(WindAxesVel), Demux/1, VelW/1, Aerodynamic Force/5, Yaw/2(WindAxesVel), Pitch/2(WindAxesVel), Roll/2(WindAxesVel), Side/2(WindAxesVel), Drag/2(WindAxesVel), Dynamic Pressure/1
  rho/1 -> Dynamic Pressure/2
  a/1 -> Wind-axes Velocities/3
  WindB/1 -> Wind-axes Velocities/2
  VelB/1 -> Wind-axes Velocities/1
  Mux/1 -> AeroCoeff/1
  CGpos/1 -> Sum1/2
  r_aero/1 -> Sum1/1
  Sum1/1 -> r x F/1
  Aerodynamic Force/1 -> Faero/1, r x F/2
  Aerodynamic Moment/1 -> Sum2/1
  Sum2/1 -> Maero/1
  r x F/1 -> Sum2/2

== system aerosimlib/FlightGear-Compatible/Complete Aircraft/CESSNA-172/Aircraft Inertia ==
  FuelFlow : Inport
  RST : Inport  Port=2
  1/2 : Gain  Gain=1/2  SaturateOnIntegerOverflow=on
  Empty Aircraft : aerosimlib/FlightGear-Compatible/Inertia/Empty Aircraft  Metrics=AC.Metrics
  Left Wing Tank : aerosimlib/FlightGear-Compatible/Propulsion/Tank/Fuel Tank  MassIni=FuelIni(1)  Tank=AC.Propulsion.Tank{1}
  Pilot Point Mass : aerosimlib/FlightGear-Compatible/Inertia/Point Mass  PointMass=AC.Metrics.PointMass{1}
  Product{,1..3} (4 alike) : Product  SaturateOnIntegerOverflow=on  InputSameDT=on
  Product4 : Product  Inputs=*/  SaturateOnIntegerOverflow=on  InputSameDT=on
  Right Wing Tank : aerosimlib/FlightGear-Compatible/Propulsion/Tank/Fuel Tank  MassIni=FuelIni(2)  Tank=AC.Propulsion.Tank{2}
  Sum1 : Sum  Inputs=++++  SaturateOnIntegerOverflow=on  InputSameDT=on
  Sum2 : Sum  Inputs=++++  SaturateOnIntegerOverflow=on  InputSameDT=on
  Sum3 : Sum  Inputs=++++  SaturateOnIntegerOverflow=on  InputSameDT=on
  Mass : Outport
  CG : Outport  Port=2
  Inertia : Outport  Port=3
  wires:
  Sum3/1 -> Inertia/1
  Right Wing Tank/3 -> Sum3/4
  Left Wing Tank/3 -> Sum3/3
  Pilot Point Mass/3 -> Sum3/2
  Empty Aircraft/3 -> Sum3/1
  Product4/1 -> CG/1
  Sum1/1 -> Product4/1
  Product2/1 -> Sum1/4
  Product1/1 -> Sum1/3
  Product/1 -> Sum1/2
  Product3/1 -> Sum1/1
  Empty Aircraft/2 -> Product3/2
  Right Wing Tank/2 -> Product2/2
  Left Wing Tank/2 -> Product1/2
  Pilot Point Mass/2 -> Product/2
  Right Wing Tank/1 -> Product2/1, Sum2/4
  Left Wing Tank/1 -> Product1/1, Sum2/3
  Pilot Point Mass/1 -> Product/1, Sum2/2
  Empty Aircraft/1 -> Product3/1, Sum2/1
  Sum2/1 -> Product4/2, Mass/1
  RST/1 -> Right Wing Tank/2, Left Wing Tank/2
  FuelFlow/1 -> 1/2/1
  1/2/1 -> Right Wing Tank/1, Left Wing Tank/1

== system aerosimlib/FlightGear-Compatible/Complete Aircraft/CESSNA-172/Atmosphere ==
  note: Inputs
  note: Outputs
  MSL : Inport  PortDimensions=1  DataType=double
  AGL : Inport  Port=2  PortDimensions=1  DataType=double
  Winds : Inport  Port=3  PortDimensions=[3 1]  DataType=double
  VelB : Inport  Port=4  PortDimensions=[3 1]  DataType=double
  VelW : Inport  Port=5  PortDimensions=[3 1]
  DCM : Inport  Port=6  PortDimensions=[3 3]  DataType=double
  Background Wind : aerosimlib/Atmosphere/Background Wind
  Standard Atmosphere : aerosimlib/Atmosphere/Standard Atmosphere
  Sum : Sum  Inputs=|++  SaturateOnIntegerOverflow=on  InputSameDT=on
  Turbulence : aerosimlib/Atmosphere/Turbulence  tsamp=tsamp
  Wind Shear : aerosimlib/Atmosphere/Wind Shear
  pstatic : Outport
  OAT : Outport  Port=2
  rho : Outport  Port=3
  a : Outport  Port=4
  WindVel : Outport  Port=5
  WindRates : Outport  Port=6
  wires:
  MSL/1 -> Standard Atmosphere/1
  Winds/1 -> Background Wind/1
  DCM/1 -> Background Wind/2
  Background Wind/1 -> Turbulence/3, Sum/2
  AGL/1 -> Turbulence/2
  VelW/1 -> Turbulence/1
  Background Wind/2 -> Wind Shear/1
  Turbulence/1 -> Sum/1
  Turbulence/2 -> Wind Shear/2
  VelB/1 -> Wind Shear/3
  Wind Shear/1 -> WindRates/1
  Standard Atmosphere/1 -> pstatic/1
  Standard Atmosphere/2 -> OAT/1
  Standard Atmosphere/3 -> rho/1
  Standard Atmosphere/4 -> a/1
  Sum/1 -> WindVel/1

== system aerosimlib/FlightGear-Compatible/Complete Aircraft/CESSNA-172/Earth ==
  note: Inputs
  note: Outputs
  Position : Inport  PortDimensions=[3 1]  DataType=double
  EGM-96 : aerosimlib/Earth/EGM-96
  Ground Alt : Constant  Value=GndAlt
  Ground Detection : aerosimlib/Earth/Ground Detection
  Mux3 : Mux  Inputs=2
  WGS-84 : aerosimlib/Earth/WGS-84
  MSL : Outport
  AGL : Outport  Port=2
  AConGnd : Outport  Port=3
  Rearth : Outport  Port=4
  Requiv : Outport  Port=5
  Gravity : Outport  Port=6
  wires:
  Position/1 -> EGM-96/1, WGS-84/1
  Ground Alt/1 -> Ground Detection/2
  EGM-96/1 -> Ground Detection/1, MSL/1
  WGS-84/1 -> Mux3/1
  WGS-84/2 -> Mux3/2
  Ground Detection/2 -> AGL/1
  Ground Detection/1 -> AConGnd/1
  Mux3/1 -> Rearth/1
  WGS-84/3 -> Requiv/1
  WGS-84/4 -> Gravity/1

== system aerosimlib/FlightGear-Compatible/Complete Aircraft/CESSNA-172/Equations of Motion ==
  note: Inputs
  note: Outputs
  Accel : Inport  PortDimensions=[3 1]
  Moment : Inport  Port=2  PortDimensions=[3 1]
  Inertia : Inport  Port=3  PortDimensions=[4 1]
  Rearth : Inport  Port=4  PortDimensions=[2 1]
  Gravity : Inport  Port=5  PortDimensions=1
  AConGnd : Inport  Port=6  PortDimensions=1
  RST : Inport  Port=7  PortDimensions=1
  Angular Rate : aerosimlib/Equations of Motion/Geodetic-Frame EOM/Angular Rate  RatesIni=RatesIni
  Attitude (Quaternions) : aerosimlib/Equations of Motion/Body-Frame EOM/Kinematics (Quaternions)  QuaternionsIni=QuaternionsIni
  Body-Inertial DCM From Quaternions : aerosimlib/Transformations/Body-Inertial DCM From Quaternions
  Demux : Demux  Outputs=2
  Euler Angles From Quaternions : aerosimlib/Transformations/Euler Angles From Quaternions
  Position : aerosimlib/Equations of Motion/Geodetic-Frame EOM/Position  PositionIni=PositionIni
  Product : Product  Multiplication=Matrix(*)  SaturateOnIntegerOverflow=on  InputSameDT=on
  Velocity : aerosimlib/Equations of Motion/Geodetic-Frame EOM/Velocity  VelocitiesIni=VelocitiesIni
  VelB : Outport
  VelNED : Outport  Port=2
  Rates : Outport  Port=3
  Quaternions : Outport  Port=4
  Pos : Outport  Port=5
  DCM : Outport  Port=6
  Euler : Outport  Port=7
  Ang Acc : Outport  Port=8
  wires:
  Attitude (Quaternions)/1 -> Quaternions/1, Euler Angles From Quaternions/1, Body-Inertial DCM From Quaternions/1
  Position/1 -> Velocity/1, Angular Rate/3, Pos/1
  Position/2 -> Velocity/2, Angular Rate/4
  Velocity/1 -> Product/2, Position/1, VelNED/1
  Demux/1 -> Position/2
  Demux/2 -> Position/3
  Rearth/1 -> Demux/1
  Gravity/1 -> Velocity/5
  RST/1 -> Velocity/6, Position/5, Angular Rate/6, Attitude (Quaternions)/2
  Angular Rate/1 -> Rates/1, Attitude (Quaternions)/1
  Moment/1 -> Angular Rate/2
  Inertia/1 -> Angular Rate/1
  Body-Inertial DCM From Quaternions/1 -> Angular Rate/5, Velocity/4, Product/1, DCM/1
  AConGnd/1 -> Position/4
  Accel/1 -> Velocity/3
  Product/1 -> VelB/1
  Angular Rate/2 -> Ang Acc/1
  Euler Angles From Quaternions/1 -> Euler/1

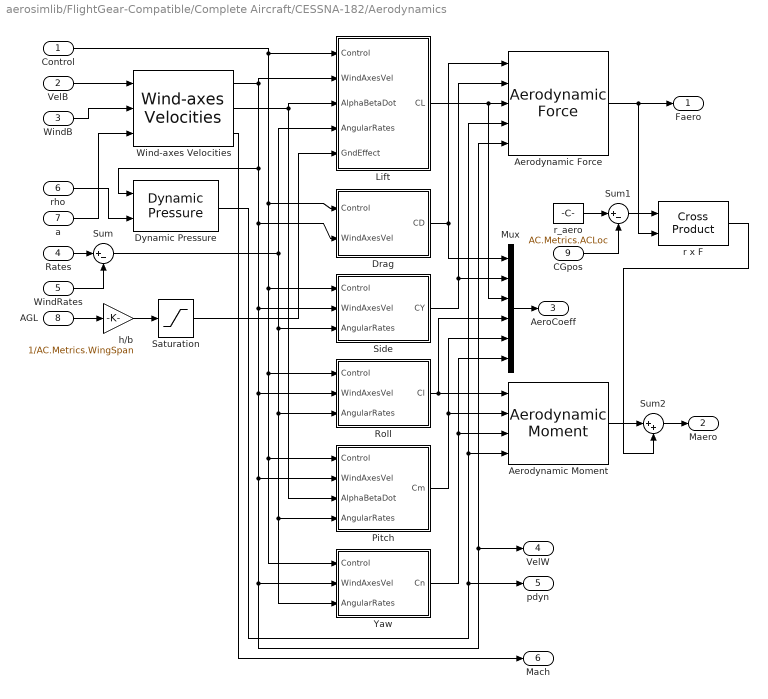
== system aerosimlib/FlightGear-Compatible/Complete Aircraft/CESSNA-182/Aerodynamics ==
  Control : Inport  PortDimensions=[4 1]
  VelB : Inport  Port=2  PortDimensions=[3 1]
  WindB : Inport  Port=3  PortDimensions=[3 1]
  Rates : Inport  Port=4  PortDimensions=[3 1]
  WindRates : Inport  Port=5  PortDimensions=[3 1]
  rho : Inport  Port=6  PortDimensions=1
  a : Inport  Port=7  PortDimensions=1
  AGL : Inport  Port=8  PortDimensions=1
  CGpos : Inport  Port=9  PortDimensions=[3 1]
  Aerodynamic Force : aerosimlib/Aerodynamics/Aerodynamic Force  S=AC.Metrics.WingArea
  Aerodynamic Moment : aerosimlib/Aerodynamics/Aerodynamic Moment  c=AC.Metrics.WingChord  b=AC.Metrics.WingSpan  S=AC.Metrics.WingArea
  Drag : Subsystem
  Dynamic Pressure : aerosimlib/Aerodynamics/Dynamic Pressure
  Lift : Subsystem
  Mux : Mux  Inputs=6
  Pitch : Subsystem
  Roll : Subsystem
  Saturation : Saturate  UpperLimit=1  LowerLimit=0
  Side : Subsystem
  Sum : Sum  Inputs=|+-  SaturateOnIntegerOverflow=on  InputSameDT=on
  Sum1 : Sum  Inputs=|+-  SaturateOnIntegerOverflow=on  InputSameDT=on
  Sum2 : Sum  Inputs=|++  SaturateOnIntegerOverflow=on  InputSameDT=on
  Wind-axes Velocities : aerosimlib/Aerodynamics/Wind-axes Velocities  Vabnd=[0 1000]  betabnd=[-1 1]  alphabnd=AC.Aerodynamics.AlphaLim
  Yaw : Subsystem
  h/b : Gain  Gain=1/AC.Metrics.WingSpan  SaturateOnIntegerOverflow=on
  r x F : aerosimlib/Math/Cross Product
  r_aero : Constant  Value=AC.Metrics.ACLoc
  Faero : Outport
  Maero : Outport  Port=2
  AeroCoeff : Outport  Port=3
  VelW : Outport  Port=4
  pdyn : Outport  Port=5
  Mach : Outport  Port=6
  wires:
  Rates/1 -> Sum/1
  Sum/1 -> Yaw/3(AngularRates), Pitch/4(AngularRates), Roll/3(AngularRates), Side/3(AngularRates), Lift/4(AngularRates)
  WindRates/1 -> Sum/2
  Saturation/1 -> Lift/5(GndEffect)
  AGL/1 -> h/b/1
  h/b/1 -> Saturation/1
  Wind-axes Velocities/3 -> Mach/1
  Aerodynamic Force/1 -> Faero/1, r x F/2
  Yaw/1(Cn) -> Mux/6, Aerodynamic Moment/3
  Pitch/1(Cm) -> Mux/5, Aerodynamic Moment/2
  Roll/1(Cl) -> Mux/4, Aerodynamic Moment/1
  Dynamic Pressure/1 -> pdyn/1, Aerodynamic Moment/4, Aerodynamic Force/4
  Side/1(CY) -> Mux/2, Aerodynamic Force/2
  Drag/1(CD) -> Mux/1, Aerodynamic Force/1
  Lift/1(CL) -> Mux/3, Aerodynamic Force/3
  Wind-axes Velocities/2 -> Lift/3(AlphaBetaDot), Pitch/3(AlphaBetaDot)
  Control/1 -> Pitch/1(Control), Yaw/1(Control), Roll/1(Control), Side/1(Control), Drag/1(Control), Lift/1(Control)
  Wind-axes Velocities/1 -> Lift/2(WindAxesVel), VelW/1, Aerodynamic Force/5, Yaw/2(WindAxesVel), Pitch/2(WindAxesVel), Roll/2(WindAxesVel), Side/2(WindAxesVel), Drag/2(WindAxesVel), Dynamic Pressure/1
  rho/1 -> Dynamic Pressure/2
  a/1 -> Wind-axes Velocities/3
  WindB/1 -> Wind-axes Velocities/2
  VelB/1 -> Wind-axes Velocities/1
  Mux/1 -> AeroCoeff/1
  CGpos/1 -> Sum1/2
  r_aero/1 -> Sum1/1
  Sum1/1 -> r x F/1
  Aerodynamic Moment/1 -> Sum2/1
  Sum2/1 -> Maero/1
  r x F/1 -> Sum2/2

== system aerosimlib/FlightGear-Compatible/Complete Aircraft/CESSNA-182/Aircraft Inertia ==
  FuelFlow : Inport
  RST : Inport  Port=2
  1/2 : Gain  Gain=1/2  SaturateOnIntegerOverflow=on
  Empty Aircraft : aerosimlib/FlightGear-Compatible/Inertia/Empty Aircraft  Metrics=AC.Metrics
  Left Wing Tank : aerosimlib/FlightGear-Compatible/Propulsion/Tank/Fuel Tank  MassIni=FuelIni(1)  Tank=AC.Propulsion.Tank{1}
  Pilot Point Mass : aerosimlib/FlightGear-Compatible/Inertia/Point Mass  PointMass=AC.Metrics.PointMass{1}
  Product{,1..3} (4 alike) : Product  SaturateOnIntegerOverflow=on  InputSameDT=on
  Product4 : Product  Inputs=*/  SaturateOnIntegerOverflow=on  InputSameDT=on
  Right Wing Tank : aerosimlib/FlightGear-Compatible/Propulsion/Tank/Fuel Tank  MassIni=FuelIni(2)  Tank=AC.Propulsion.Tank{2}
  Sum1 : Sum  Inputs=++++  SaturateOnIntegerOverflow=on  InputSameDT=on
  Sum2 : Sum  Inputs=++++  SaturateOnIntegerOverflow=on  InputSameDT=on
  Sum3 : Sum  Inputs=++++  SaturateOnIntegerOverflow=on  InputSameDT=on
  Mass : Outport
  CG : Outport  Port=2
  Inertia : Outport  Port=3
  wires:
  Sum3/1 -> Inertia/1
  Right Wing Tank/3 -> Sum3/4
  Left Wing Tank/3 -> Sum3/3
  Pilot Point Mass/3 -> Sum3/2
  Empty Aircraft/3 -> Sum3/1
  Product4/1 -> CG/1
  Sum1/1 -> Product4/1
  Product2/1 -> Sum1/4
  Product1/1 -> Sum1/3
  Product/1 -> Sum1/2
  Product3/1 -> Sum1/1
  Empty Aircraft/2 -> Product3/2
  Right Wing Tank/2 -> Product2/2
  Left Wing Tank/2 -> Product1/2
  Pilot Point Mass/2 -> Product/2
  Right Wing Tank/1 -> Product2/1, Sum2/4
  Left Wing Tank/1 -> Product1/1, Sum2/3
  Pilot Point Mass/1 -> Product/1, Sum2/2
  Empty Aircraft/1 -> Product3/1, Sum2/1
  Sum2/1 -> Product4/2, Mass/1
  RST/1 -> Right Wing Tank/2, Left Wing Tank/2
  FuelFlow/1 -> 1/2/1
  1/2/1 -> Right Wing Tank/1, Left Wing Tank/1

== system aerosimlib/FlightGear-Compatible/Complete Aircraft/CESSNA-182/Earth ==
  note: Inputs
  note: Outputs
  Position : Inport  PortDimensions=[3 1]  DataType=double
  EGM-96 : aerosimlib/Earth/EGM-96
  Ground Alt : Constant  Value=GndAlt
  Ground Detection : aerosimlib/Earth/Ground Detection
  Mux3 : Mux  Inputs=2
  WGS-84 : aerosimlib/Earth/WGS-84
  MSL : Outport
  AGL : Outport  Port=2
  AConGnd : Outport  Port=3
  Rearth : Outport  Port=4
  Requiv : Outport  Port=5
  Gravity : Outport  Port=6
  wires:
  Position/1 -> EGM-96/1, WGS-84/1
  Ground Alt/1 -> Ground Detection/2
  EGM-96/1 -> Ground Detection/1, MSL/1
  WGS-84/1 -> Mux3/1
  WGS-84/2 -> Mux3/2
  Ground Detection/2 -> AGL/1
  Ground Detection/1 -> AConGnd/1
  Mux3/1 -> Rearth/1
  WGS-84/3 -> Requiv/1
  WGS-84/4 -> Gravity/1
